simulink model "ex4"  (R2015a)
settings: Solver=ode3  StartTime=0.0  StopTime=0.05  FixedStep=2e-5  RelTol=1e-3
undefined symbols (not defined in the file or in its folder): gcbh, rcfiltgaincompat
libraries: simulink x2, commfilt2 x2, commchan3 x1, dsparch4 x1, commsink2 x1, commrandsrc2 x1, dspsigops x1
settings Model: Creator=ctu  LastModifiedBy=ctu

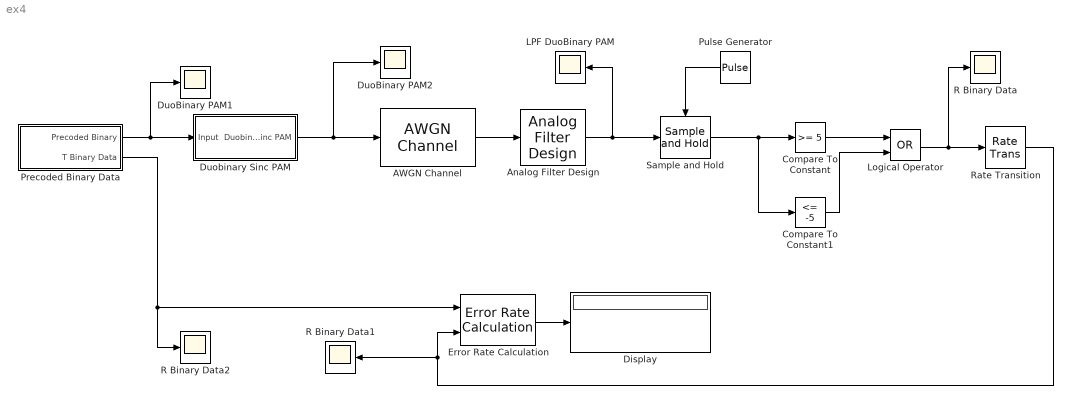
== system ex4 ==
  AWGN Channel : commchan3/AWGN Channel  InputProcessing=Inherited (this choice will be removed - see release notes)  seed=randseed  noiseMode=Variance from mask  EbNodB=10  EsNodB=10  SNRdB=10  bitsPerSym=1  Ps=1  Tsym=1  variance=10
  Analog Filter Design : dsparch4/Analog Filter Design  method=Chebyshev I  filttype=Lowpass  N=9  Wlo=2*pi*600  Whi=80  Rp=0.1  Rs=40
  Compare To Constant : simulink/Logic and Bit Operations/Compare To Constant  relop=>=  const=5  OutDataTypeStr=boolean
  Compare To Constant1 : simulink/Logic and Bit Operations/Compare To Constant  relop=<=  const=-5  OutDataTypeStr=boolean
  Display : Display
      settings: Decimation=3
  DuoBinary PAM1 : Scope
      settings: YMin=-1.5  YMax=1.5
  DuoBinary PAM2 : Scope
      settings: SaveName=ScopeData5
  Duobinary Sinc PAM : Subsystem
  Error Rate Calculation : commsink2/Error Rate Calculation  N=8  st_delay=2  cp_mode=Entire frame  subframe=[]  PMode=Port  WsName=ErrorVec  RsMode2=off  stop=off  numErr=100  maxBits=1e6
  LPF DuoBinary PAM : Scope
      settings: YMin=-15  YMax=15  SaveName=ScopeData6
  Logical Operator : Logic  Operator=OR  AllPortsSameDT=off  OutDataTypeStr=boolean
  Precoded Binary Data : Subsystem
  Pulse Generator : DiscretePulseGenerator  PulseType=Time based  Period=1e-3  PulseWidth=2
  R Binary Data : Scope
      settings: YMin=-0.5  YMax=1.5  SaveName=ScopeData7
  R Binary Data1 : Scope
      settings: YMin=-0.5  YMax=1.5  SaveName=ScopeData4
  R Binary Data2 : Scope
      settings: YMin=-0.5  YMax=1.5  SaveName=ScopeData3
  Rate Transition : RateTransition  OutPortSampleTime=1e-3
  Sample and Hold : dspsigops/Sample and Hold  trig=Rising edge  initCond=0  latchinput=off
  wires:
  Duobinary Sinc PAM/1(Duobinary Sinc PAM) -> DuoBinary PAM2/1, AWGN Channel/1
  AWGN Channel/1 -> Analog Filter Design/1
  Analog Filter Design/1 -> LPF DuoBinary PAM/1, Sample and Hold/1
  Pulse Generator/1 -> Sample and Hold/Trigger
  Sample and Hold/1 -> Compare To Constant1/1, Compare To Constant/1
  Compare To Constant/1 -> Logical Operator/1
  Compare To Constant1/1 -> Logical Operator/2
  Logical Operator/1 -> R Binary Data/1, Rate Transition/1
  Error Rate Calculation/1 -> Display/1
  Rate Transition/1 -> Error Rate Calculation/2, R Binary Data1/1
  Precoded Binary Data/1(Precoded Binary) -> DuoBinary PAM1/1, Duobinary Sinc PAM/1(Input)
  Precoded Binary Data/2(T Binary Data) -> R Binary Data2/1, Error Rate Calculation/1

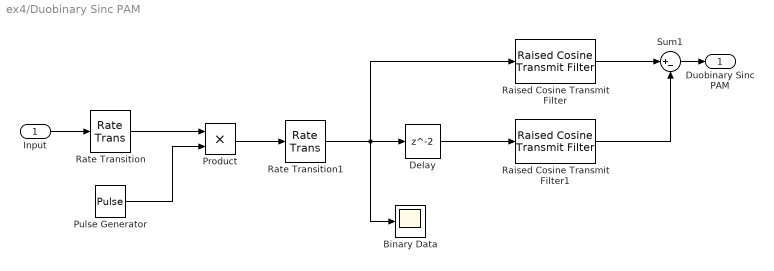
== system ex4/Duobinary Sinc PAM ==
  Input : Inport
  Binary Data : Scope
      settings: YMin=-1.5  YMax=1.5  SaveName=ScopeData2
  Delay : Delay  InitialCondition=0  InputProcessing=Inherited
  Product : Product
  Pulse Generator : DiscretePulseGenerator  PulseType=Time based  Period=1e-3  PulseWidth=2
  Raised Cosine Transmit Filter : commfilt2/Raised Cosine Transmit Filter  filtType=Normal  filtSpan=8  currentFiltSpan=8  D=(8)/2  R=0  sampMode=Mute  saveAsFlag=0  N=50  framing=Allow multirate processing  InputProcessing=Inherited (this choice will be removed - see release notes)  checkGain=Normalized  filterGain=(5)*rcfiltgaincompat(gcbh)  checkCoeff=off  variableName=rcTxFilt  launchFVT=on  roundingMode=Floor  overflowMode=off
  Raised Cosine Transmit Filter1 : commfilt2/Raised Cosine Transmit Filter  filtType=Normal  filtSpan=8  currentFiltSpan=8  D=(8)/2  R=0  sampMode=Mute  saveAsFlag=0  N=50  framing=Allow multirate processing  InputProcessing=Inherited (this choice will be removed - see release notes)  checkGain=Normalized  filterGain=(5)*rcfiltgaincompat(gcbh)  checkCoeff=off  variableName=rcTxFilt1  launchFVT=on  roundingMode=Floor  overflowMode=off
  Rate Transition : RateTransition  OutPortSampleTime=2e-5
  Rate Transition1 : RateTransition  OutPortSampleTime=1e-3
  Sum1 : Sum  Inputs=|+-
  Duobinary Sinc PAM : Outport
  wires:
  Rate Transition/1 -> Product/1
  Pulse Generator/1 -> Product/2
  Product/1 -> Rate Transition1/1
  Sum1/1 -> Duobinary Sinc PAM/1
  Rate Transition1/1 -> Delay/1, Binary Data/1, Raised Cosine Transmit Filter/1
  Delay/1 -> Raised Cosine Transmit Filter1/1
  Raised Cosine Transmit Filter1/1 -> Sum1/2
  Raised Cosine Transmit Filter/1 -> Sum1/1
  Input/1 -> Rate Transition/1

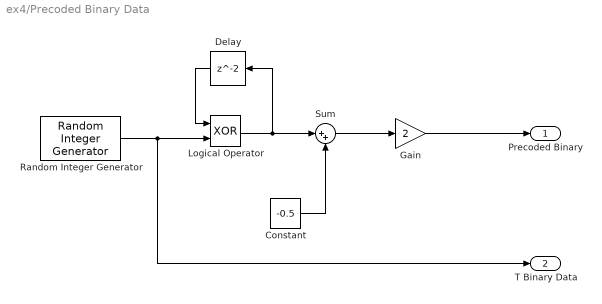
== system ex4/Precoded Binary Data ==
  Constant : Constant  Value=-0.5
  Delay : Delay  InitialCondition=0  InputProcessing=Inherited
  Gain : Gain  Gain=2
  Logical Operator : Logic  Operator=XOR  AllPortsSameDT=off  OutDataTypeStr=boolean
  Random Integer Generator : commrandsrc2/Random Integer Generator  mul=2  seed=randseed  Ts=1e-3  frameBased=off  sampPerFrame=1  orient=off  outDataType=boolean
  Sum : Sum  Inputs=|++
  Precoded Binary : Outport
  T Binary Data : Outport  Port=2
  wires:
  Random Integer Generator/1 -> T Binary Data/1, Logical Operator/2
  Delay/1 -> Logical Operator/1
  Logical Operator/1 -> Delay/1, Sum/1
  Constant/1 -> Sum/2
  Sum/1 -> Gain/1
  Gain/1 -> Precoded Binary/1
